simulink model "hummingbird"  (R2018a)
settings: Solver=FixedStepAuto  StartTime=0.0  StopTime=inf  FixedStep=0.01  RelTol=1e-3
InitFcn:
  | loadRobot
model workspace (MAT data in the model file):
  SL_ROS_VariableLengthArrays_MaxSizes.CommonInfo.ArrayTruncateAction = 'EmitWarning'
  SL_ROS_VariableLengthArrays_MaxSizes.MsgTypeMap = containers.Map
  SL_ROS_VariableLengthArrays_MaxSizes.MsgTypeMap.serialization.keys = {'sensor_msgs/Image'}
  SL_ROS_VariableLengthArrays_MaxSizes.MsgTypeMap.serialization.values{1}(1).PropertyName = 'Data'
  SL_ROS_VariableLengthArrays_MaxSizes.MsgTypeMap.serialization.values{1}(1).DataType = 'uint8'
  SL_ROS_VariableLengthArrays_MaxSizes.MsgTypeMap.serialization.values{1}(1).MaxLength = 921600
  SL_ROS_VariableLengthArrays_MaxSizes.MsgTypeMap.serialization.values{1}(2).PropertyName = 'Encoding'
  SL_ROS_VariableLengthArrays_MaxSizes.MsgTypeMap.serialization.values{1}(2).DataType = 'uint8'
  SL_ROS_VariableLengthArrays_MaxSizes.MsgTypeMap.serialization.values{1}(2).MaxLength = 128
  SL_ROS_VariableLengthArrays_MaxSizes.MsgTypeMap.serialization.uniformity = 0
  SL_ROS_VariableLengthArrays_MaxSizes.MsgTypeMap.serialization.keyType = 'char'
  SL_ROS_VariableLengthArrays_MaxSizes.MsgTypeMap.serialization.valueType = 'any'
values from neighbouring files (symbols this model uses):
  minRot = 30    [loadRobot.m]
  minTrackRot = 10    [loadRobot.m]
  minTrackTrans = 0.2    [loadRobot.m]
  minTrans = 1    [loadRobot.m]
  sampleTime = 0.01    [loadRobot.m]
undefined symbols (not defined in the file or in its folder): Pose, W, X, Y, Z
libraries: robotlib x9, hummingbirdLibrary x4, robotcorelib x1
settings Model: Creator=scastro  LastModifiedBy=vuwij
settings OptimizationCC: PassReuseOutputArgsAs=Individual arguments  MaxStackSize=64
settings DebuggingCC: ParameterTunabilityLossMsg=error
settings HardwareCC: ProdBitPerPointer=32  ProdBitPerSizeT=32  ProdBitPerPtrDiffT=32  ProdLargestAtomicFloat=None  ProdIntDivRoundTo=Undefined  ProdEndianess=Unspecified  ProdWordSize=32  ProdHWDeviceType=Generic->Unspecified (assume 32-bit Generic)
settings SFSimCC: MATLABDynamicMemAlloc=off
settings RTWCC: SystemTargetFile=ert.tlc  HardwareBoard=Robot Operating System (ROS)  TLCOptions="-aInlineSetEventsForThisBaseRateFcn=TLC_FALSE -aSuppressMultiTaskScheduler=TLC_FALSE  -aRateBasedStepFcn=0"  TemplateMakefile=ert_default_tmf  GenerateReport=on  Toolchain=Catkin  IncludeHyperlinkInReport=on  LaunchReport=on  TargetLang=C++  GenerateTraceInfo=on  GenerateTraceReport=on  GenerateTraceReportSl=on  GenerateTraceReportSf=on  GenerateTraceReportEml=on
settings CodeAppCC: ForceParamTrailComments=on  IgnoreCustomStorageClasses=off  OperatorAnnotations=on  SimulinkDataObjDesc=on  SFDataObjDesc=on  InsertBlockDesc=on
settings ERTTargetCC: SupportVariableSizeSignals=on

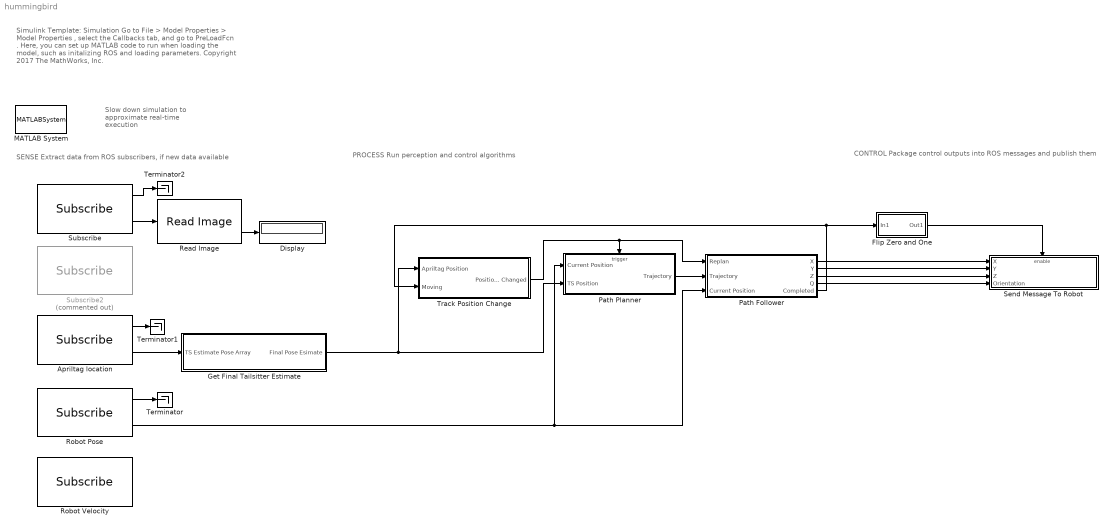
== system hummingbird ==
  note: Simulink Template: Simulation
      |
      | Go to File > Model Properties > Model Properties , select the Callbacks tab, and go to PreLoadFcn .
      |
      | Here, you can set up MATLAB code to run when loading the model, such as initalizing ROS and loading parameters.
      |
      | Copyright 2017 The MathWorks, Inc.
  note: Slow down simulation to approximate real-time execution
  note: PROCESS
      | Run perception and control algorithms
  note: SENSE
      | Extract data from ROS subscribers, if new data available
  note: CONTROL
      | Package control outputs into ROS messages and publish them
  Apriltag location : robotlib/Subscribe  SourceLibraryInfo=This block requires Robotics System Toolbox  topicSource=Select from ROS network  topic=/ts_location_estimates  messageType=geometry_msgs/PoseArray  sampleTime=-1  messageQueueLength=1
      settings: SourceProductBaseCode=RO
  Display : Display
  Flip Zero and One : Subsystem
  Get Final Tailsitter Estimate : Subsystem
  MATLAB System : MATLABSystem  System=ExampleHelperSimulationRateControl  SampleTime=sampleTime
      mask Type: ExampleHelperSimulationRateControl
      mask Display: disp('Rate Control');
  Path Follower : Subsystem
  Path Planner : Subsystem  TreatAsAtomicUnit=on
  Read Image : robotlib/Read Image  SourceLibraryInfo=This block requires Robotics System Toolbox  MaximumImageSize=[ 480, 640 ]  ImageEncoding=rgb8  ShowAlphaOutput=off  ShowErrorCodeOutput=on  VariableSizeOutputs=off
      settings: SourceProductName=Robotics System Toolbox  SourceProductBaseCode=RO
  Robot Pose : robotlib/Subscribe  SourceLibraryInfo=This block requires Robotics System Toolbox  topicSource=Select from ROS network  topic=/mavros/global_position/local  messageType=nav_msgs/Odometry  sampleTime=-1  messageQueueLength=1
      settings: SourceProductBaseCode=RO
  Robot Velocity : robotlib/Subscribe  SourceLibraryInfo=This block requires Robotics System Toolbox  topicSource=Select from ROS network  topic=/mavros/local_position/velocity  messageType=geometry_msgs/TwistStamped  sampleTime=-1  messageQueueLength=1
      settings: SourceProductBaseCode=RO
  Send Message To Robot : Subsystem
  Subscribe : robotlib/Subscribe  SourceLibraryInfo=This block requires Robotics System Toolbox  topicSource=Select from ROS network  topic=/camera/color/image_raw  messageType=sensor_msgs/Image  sampleTime=-1  messageQueueLength=1
      settings: SourceProductBaseCode=RO
  Subscribe2 : robotlib/Subscribe  Commented=on  SourceLibraryInfo=This block requires Robotics System Toolbox  topicSource=Select from ROS network  topic=/tag_detections_image  messageType=sensor_msgs/Image  sampleTime=-1  messageQueueLength=1
      settings: SourceProductBaseCode=RO
  Terminator : Terminator
  Terminator1 : Terminator
  Terminator2 : Terminator
  Track Position Change : Subsystem
  wires:
  Read Image/2 -> Display/1
  Subscribe/2 -> Read Image/1
  Path Planner/1(Trajectory) -> Path Follower/2(Trajectory)
  Track Position Change/1(Position Changed) -> Path Follower/1(Replan), Path Planner/Trigger
  Robot Pose/1 -> Terminator/1
  Apriltag location/1 -> Terminator1/1
  Subscribe/1 -> Terminator2/1
  Path Follower/5(Completed) -> Track Position Change/2(Moving), Flip Zero and One/1(In1)
  Flip Zero and One/1(Out1) -> Send Message To Robot/Enable
  Apriltag location/2 -> Get Final Tailsitter Estimate/1(TS Estimate Pose Array)
  Path Follower/1(X) -> Send Message To Robot/1(X)
  Path Follower/2(Y) -> Send Message To Robot/2(Y)
  Path Follower/3(Z) -> Send Message To Robot/3(Z)
  Path Follower/4(Q) -> Send Message To Robot/4(Orientation)
  Robot Pose/2 -> Path Follower/3(Current Position), Path Planner/1(Current Position)
  Get Final Tailsitter Estimate/1(Final Pose Esimate) -> Track Position Change/1(Apriltag Position), Path Planner/2(TS Position)

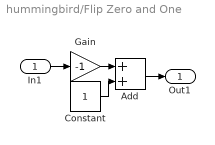
== system hummingbird/Flip Zero and One ==
  In1 : Inport
  Add : Sum
  Constant : Constant
  Gain : Gain  Gain=-1
  Out1 : Outport
  wires:
  Constant/1 -> Add/2
  Add/1 -> Out1/1
  In1/1 -> Gain/1
  Gain/1 -> Add/1

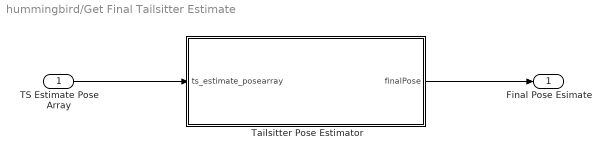
== system hummingbird/Get Final Tailsitter Estimate ==
  TS Estimate Pose Array : Inport
  Tailsitter Pose Estimator : MATLAB Function  TreatAsAtomicUnit=on
  Final Pose Esimate : Outport
  wires:
  TS Estimate Pose Array/1 -> Tailsitter Pose Estimator/1(ts_estimate_posearray)
  Tailsitter Pose Estimator/1(finalPose) -> Final Pose Esimate/1

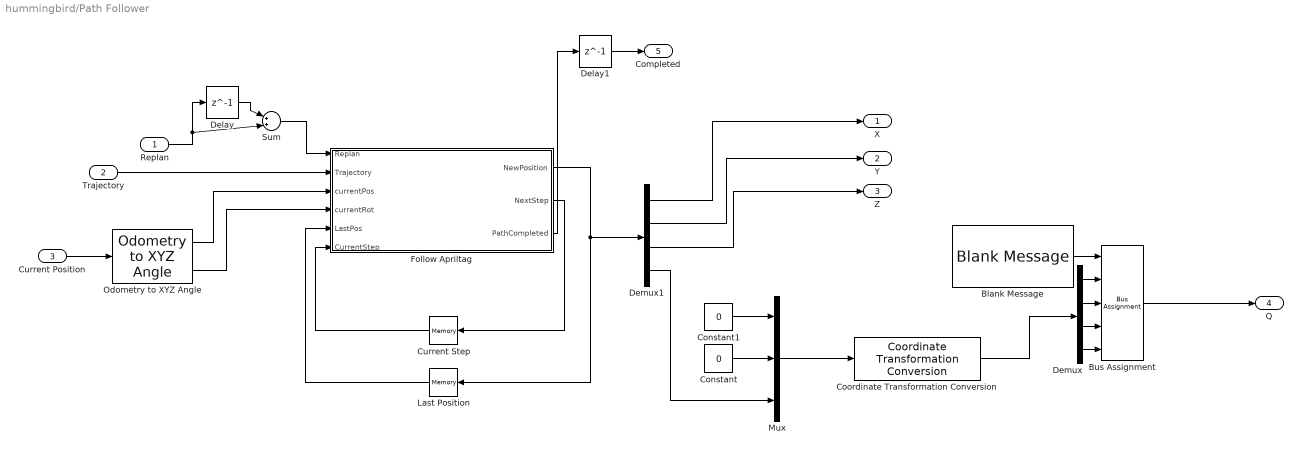
== system hummingbird/Path Follower ==
  Replan : Inport
  Trajectory : Inport  Port=2  SampleTime=0.01
      settings: VarSizeSig=Yes
  Current Position : Inport  Port=3
  Blank Message : robotlib/Blank Message  SourceLibraryInfo=This block requires Robotics System Toolbox  messageType=geometry_msgs/Quaternion  SampleTime=-1
      settings: SourceProductBaseCode=RO
  Bus Assignment : BusAssignment  AssignedSignals=X,Y,Z,W
  Constant : Constant  Value=0
  Constant1 : Constant  Value=0
  Coordinate Transformation Conversion : robotcorelib/Coordinate Transformation Conversion  InputRepresentation=Euler Angles  InputEulerSequence=ZYX  ShowTrVecInputPort=on  OutputRepresentation=Quaternion  OutputEulerSequence=ZYX  ShowTrVecOutputPort=on  SimulateUsing=Interpreted execution
      settings: SourceProductBaseCode=RO
  Current Step : Memory  InitialCondition=1
  Delay : Delay  DelayLength=1
  Delay1 : Delay  DelayLength=1  InitialCondition=1
  Demux : Demux
  Demux1 : Demux
  Follow Apriltag : MATLAB Function  TreatAsAtomicUnit=on
  Last Position : Memory  InitialCondition=[0,0,0,0]
  Mux : Mux  Inputs=3
  Odometry to XYZ Angle : hummingbirdLibrary/Odometry to XYZ Angle
  Sum : Sum  Inputs=|++|
  X : Outport
  Y : Outport  Port=2
  Z : Outport  Port=3
  Q : Outport  Port=4
  Completed : Outport  Port=5
  wires:
  Follow Apriltag/2(NextStep) -> Current Step/1
  Current Step/1 -> Follow Apriltag/6(CurrentStep)
  Replan/1 -> Sum/2, Delay/1
  Last Position/1 -> Follow Apriltag/5(LastPos)
  Blank Message/1 -> Bus Assignment/1
  Bus Assignment/1 -> Q/1
  Demux/1 -> Bus Assignment/2
  Demux/3 -> Bus Assignment/4
  Demux/4 -> Bus Assignment/5
  Demux/2 -> Bus Assignment/3
  Coordinate Transformation Conversion/1 -> Demux/1
  Constant1/1 -> Mux/1
  Constant/1 -> Mux/2
  Mux/1 -> Coordinate Transformation Conversion/1
  Demux1/4 -> Mux/3
  Current Position/1 -> Odometry to XYZ Angle/1
  Odometry to XYZ Angle/1 -> Follow Apriltag/3(currentPos)
  Odometry to XYZ Angle/2 -> Follow Apriltag/4(currentRot)
  Trajectory/1 -> Follow Apriltag/2(Trajectory)
  Demux1/1 -> X/1
  Demux1/2 -> Y/1
  Demux1/3 -> Z/1
  Follow Apriltag/3(PathCompleted) -> Delay1/1
  Delay1/1 -> Completed/1
  Delay/1 -> Sum/1
  Sum/1 -> Follow Apriltag/1(Replan)
  Follow Apriltag/1(NewPosition) -> Demux1/1, Last Position/1

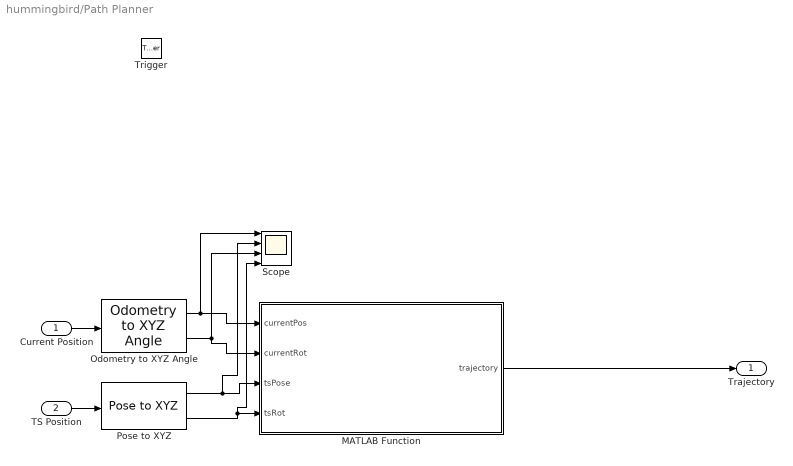
== system hummingbird/Path Planner ==
  Current Position : Inport
  TS Position : Inport  Port=2
  Trigger : TriggerPort  VariantControl=Variant  InitialTriggerSignalState=zero
  MATLAB Function : MATLAB Function  TreatAsAtomicUnit=on
  Odometry to XYZ Angle : hummingbirdLibrary/Odometry to XYZ Angle
  Pose to XYZ : hummingbirdLibrary/Pose to XYZ
  Scope : Scope  NumInputPorts=4
  Trajectory : Outport
  wires:
  MATLAB Function/1(trajectory) -> Trajectory/1
  TS Position/1 -> Pose to XYZ/1
  Odometry to XYZ Angle/2 -> MATLAB Function/2(currentRot), Scope/3
  Odometry to XYZ Angle/1 -> Scope/1, MATLAB Function/1(currentPos)
  Pose to XYZ/1 -> Scope/2, MATLAB Function/3(tsPose)
  Pose to XYZ/2 -> Scope/4, MATLAB Function/4(tsRot)
  Current Position/1 -> Odometry to XYZ Angle/1

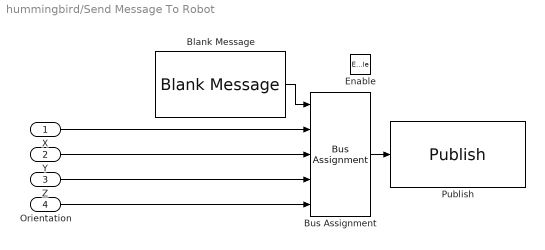
== system hummingbird/Send Message To Robot ==
  X : Inport
  Y : Inport  Port=2
  Z : Inport  Port=3
  Orientation : Inport  Port=4
  Enable : EnablePort
  Blank Message : robotlib/Blank Message  SourceLibraryInfo=This block requires Robotics System Toolbox  messageType=geometry_msgs/PoseStamped  SampleTime=-1
      settings: SourceProductBaseCode=RO
  Bus Assignment : BusAssignment  AssignedSignals=Pose.Position.X,Pose.Position.Y,Pose.Position.Z,Pose.Orientation
  Publish : robotlib/Publish  SourceLibraryInfo=This block requires Robotics System Toolbox  topicSource=Select from ROS network  topic=/mavros/setpoint_position/local  messageType=geometry_msgs/PoseStamped  messageQueueLength=1
      settings: SourceProductBaseCode=RO
  wires:
  X/1 -> Bus Assignment/2
  Y/1 -> Bus Assignment/3
  Orientation/1 -> Bus Assignment/5
  Z/1 -> Bus Assignment/4
  Bus Assignment/1 -> Publish/1
  Blank Message/1 -> Bus Assignment/1

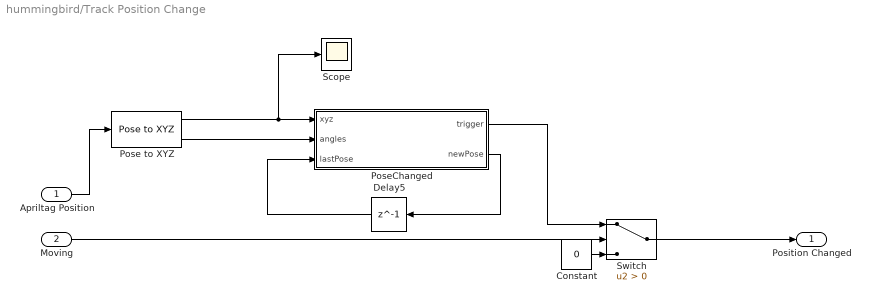
== system hummingbird/Track Position Change ==
  Apriltag Position : Inport
  Moving : Inport  Port=2
  Constant : Constant  Value=0
  Delay5 : Delay  DelayLength=1  InitialCondition=[0 0 0 0]  UseCircularBuffer=on
  Pose to XYZ : hummingbirdLibrary/Pose to XYZ
  PoseChanged : MATLAB Function  TreatAsAtomicUnit=on
  Scope : Scope
  Switch : Switch  Criteria=u2 > Threshold
  Position Changed : Outport  PortDimensions=1
  wires:
  PoseChanged/2(newPose) -> Delay5/1
  Apriltag Position/1 -> Pose to XYZ/1
  PoseChanged/1(trigger) -> Switch/1
  Pose to XYZ/1 -> Scope/1, PoseChanged/1(xyz)
  Pose to XYZ/2 -> PoseChanged/2(angles)
  Delay5/1 -> PoseChanged/3(lastPose)
  Moving/1 -> Switch/2
  Constant/1 -> Switch/3
  Switch/1 -> Position Changed/1

== matlab function hummingbird/Track Position Change/PoseChanged ==
  data: trigger output; xyz input; angles input; newPose output; lastPose input size=[1,4]; minTrans parameter; minRot parameter
function [trigger, newPose] = PoseChanged(xyz, angles, lastPose, minTrans, minRot)
    x = xyz(1);
    y = xyz(2);
    z = xyz(3);
    yaw = rad2deg(angles(1));
    
    poseTranslated = [x y z yaw];
    
    newPose = lastPose;
    
    if(norm(lastPose(1,1:3) - poseTranslated(1,1:3)) > minTrans || abs(lastPose(4) - poseTranslated(4)) > minRot)
        newPose(1,1:4) = poseTranslated;
        trigger = 1;
    else
        trigger = 0;
    end
end

== matlab function hummingbird/Path Planner/MATLAB Function ==
  data: currentPos input; trajectory output size=[10000,4]; currentRot input; tsPose input; tsRot input
function trajectory = find_path_to_tailsitter(currentPos, currentRot, tsPose, tsRot)
    trajectory = tailsitter_bezier_path(currentPos, currentRot, tsPose, tsRot, 0.2);
    plot3(trajectory(:,1), trajectory(:,2), trajectory(:,3));
    grid minor;
end

== matlab function hummingbird/Path Follower/Follow Apriltag ==
  data: NewPosition output; Replan input; Trajectory input; currentPos input; currentRot input; LastPos input size=[1,4]; CurrentStep input; NextStep output; minTrackRot parameter; minTrackTrans parameter; PathCompleted output
function [NewPosition, NextStep, PathCompleted] = FollowObject(Replan, Trajectory, currentPos, currentRot, LastPos, CurrentStep, minTrackRot, minTrackTrans)

    Xcur = currentPos(1);
    Ycur = currentPos(2);
    Zcur = currentPos(3);
    Yawcur = currentRot(1);
    
    % Set the new position
    NewPosition = LastPos;
    if(isequal(LastPos, [0,0,0,0])) 
        NewPosition = [Xcur Ycur Zcur Yawcur];
    else
        NewPosition(1,1:4) = LastPos;
    end
    
    if(Replan == 1)
        NextStep = 1;
        PathCompleted = 0;
        return;
    end
    
    % Follow a trajectory if there is one
    [l, ~] = size(Trajectory);
    if(l ~= 0)
        if (CurrentStep < l)
            NextStep = CurrentStep + 1;
            NewPosition(1,1:4) = Trajectory(NextStep,:);
            PathCompleted = 0;
        else
            NextStep = CurrentStep;
            PathCompleted = 1;
            NewPosition(1,1:4) = LastPos;
        end
    else
        NextStep = 1;
        PathCompleted = 1;
    end
end

== matlab function hummingbird/Get Final Tailsitter Estimate/Tailsitter Pose Estimator ==
  data: ts_estimate_posearray input Bus: SL_Bus_hummingbird_geometry_msgs_PoseArray; finalPose output Bus: SL_Bus_hummingbird_geometry_msgs_Pose
function finalPose = TailsitterPoseEstimator(ts_estimate_posearray)
    % Average Only, then set first one to average
    finalPose = ts_estimate_posearray.Poses(1);
    
    count = 1;
    for i = 1:4
        if(ts_estimate_posearray.Poses(i).Position.X ~= 0 || ts_estimate_posearray.Poses(i).Position.Y ~= 0 || ts_estimate_posearray.Poses(i).Position.Z ~= 0)
            ts_estimate_posearray.Poses(1).Position.X = ts_estimate_posearray.Poses(1).Position.X + ts_estimate_posearray.Poses(i).Position.X;
            ts_estimate_posearray.Poses(1).Position.Y = ts_estimate_posearray.Poses(1).Position.Y + ts_estimate_posearray.Poses(i).Position.Y;
            ts_estimate_posearray.Poses(1).Position.Z = ts_estimate_posearray.Poses(1).Position.Z + ts_estimate_posearray.Poses(i).Position.Z;
            count = count + 1;
        end
    end
    
    ts_estimate_posearray.Poses(1).Position.X = ts_estimate_posearray.Poses(1).Position.X / count;
    ts_estimate_posearray.Poses(1).Position.Y = ts_estimate_posearray.Poses(1).Position.Y / count;
    ts_estimate_posearray.Poses(1).Position.Z = ts_estimate_posearray.Poses(1).Position.Z / count;
    
end
